simulink model "two_tanks_model_cascade"  (R2018b)
settings: Solver=FixedStepAuto  StartTime=0.0  StopTime=2400  FixedStep=0.1  RelTol=1e-3
model workspace (MATLAB code in the model file):
  | A1 = 1;
  | a1 = 0.1*0.1;
  | A2 = A1;
  | a2 = a1;
  | h10 = 1;
  | h20=1;
values from neighbouring files (symbols this model uses):
  K = yf/uf    (= 58.7333333333)    [two_tanks_cascade.m]    (also in two_tanks_cascade_ffwd.m)
  kc1 = 0.406    [two_tanks_cascade.m]    (also in two_tanks_cascade_ffwd.m)
  kc2 = 1    [two_tanks_cascade.m]    (also in two_tanks_cascade_ffwd.m)
  tau = 59    [two_tanks_cascade.m]    (also in two_tanks_cascade_ffwd.m)
  taui1 = t1/z1    (= 8.96)    [two_tanks_cascade.m]    (also in two_tanks_cascade_ffwd.m)
  taui2 = t2    (= 59)    [two_tanks_cascade.m]    (also in two_tanks_cascade_ffwd.m)
undefined symbols (not defined in the file or in its folder): theta
settings Model: PacingRate=100  Creator=kjartan  LastModifiedBy=kjartan

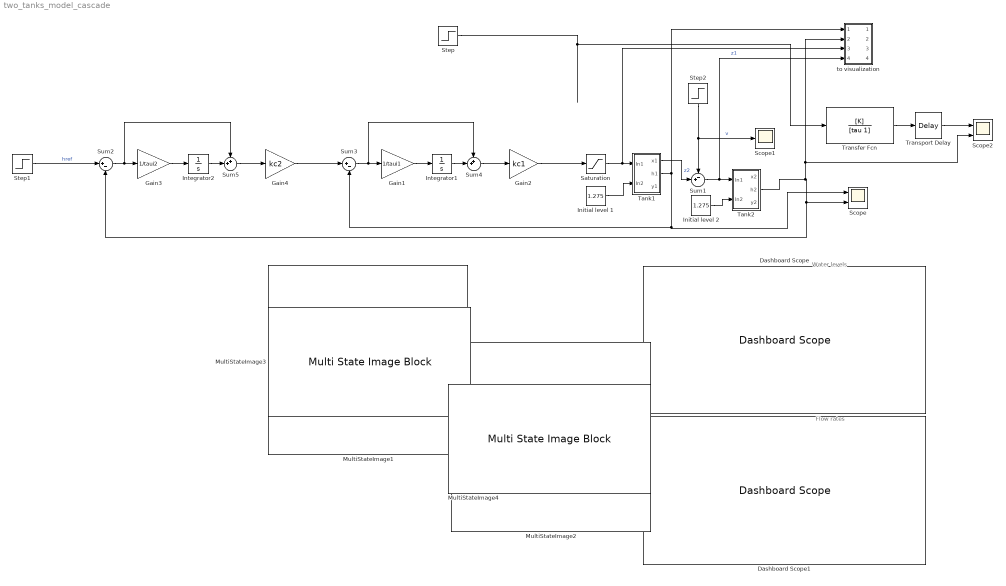
== system two_tanks_model_cascade ==
  note: Flow rates
  note: Water levels
  Dashboard Scope : DashboardScope  WebBlockId=50  Ymin=0  Ymax=2.6000000000000001
  Dashboard Scope1 : DashboardScope  WebBlockId=91  Ymin=0  Ymax=0.29999999999999999
  Gain1 : Gain  Gain=1/taui1
  Gain2 : Gain  Gain=kc1
  Gain3 : Gain  Gain=1/taui2
  Gain4 : Gain  Gain=kc2
  Initial level 1 : Constant  Value=1.275
  Initial level 2 : Constant  Value=1.275
  Integrator1 : Integrator
  Integrator2 : Integrator
  MultiStateImage1 : MultiStateImageBlock  WebBlockId=71
  MultiStateImage2 : MultiStateImageBlock  WebBlockId=119
  MultiStateImage3 : MultiStateImageBlock  WebBlockId=117  ScaleMode=Fill
  MultiStateImage4 : MultiStateImageBlock  WebBlockId=126  ScaleMode=Fill
  Saturation : Saturate  LowerLimit=0
  Scope : Scope  NumInputPorts=2
  Scope1 : Scope
  Scope2 : Scope  NumInputPorts=2
  Step : Step  Time=800  Before=0.05  After=0.065  SampleTime=0
  Step1 : Step  Time=800  Before=1.275  After=2  SampleTime=0
  Step2 : Step  Time=1400  After=0.015  SampleTime=0
  Sum1 : Sum  Inputs=-+|
  Sum2 : Sum  Inputs=|+-
  Sum3 : Sum  Inputs=|+-
  Sum4 : Sum  Inputs=++|
  Sum5 : Sum  Inputs=++|
  Tank1 : Subsystem
  Tank2 : Subsystem
  Transfer Fcn : TransferFcn  Numerator=[K]  Denominator=[tau 1]
  Transport Delay : TransportDelay  DelayTime=theta
  to visualization : Subsystem
  wires:
  Tank1/1(x1) -> Sum1/2  "z2"
  Tank1/2(h1) -> to visualization/1(In2), Sum3/2, Scope/1
  Sum1/1 -> to visualization/4(In4), Tank2/1(In1)
  Step1/1 -> Sum2/1  "href"
  Saturation/1 -> to visualization/3(In3), Tank1/1(In1)  "z1"
  Initial level 2/1 -> Tank2/2(In2)
  Initial level 1/1 -> Tank1/2(In2)
  Step2/1 -> Sum1/1, Scope1/1  "v"
  Step/1 -> Transfer Fcn/1
  Transfer Fcn/1 -> Transport Delay/1
  Transport Delay/1 -> Scope2/1
  Gain1/1 -> Integrator1/1
  Integrator1/1 -> Sum4/2
  Sum3/1 -> Sum4/1, Gain1/1
  Sum4/1 -> Gain2/1
  Gain2/1 -> Saturation/1
  Gain3/1 -> Integrator2/1
  Tank2/2(h2) -> Scope2/2, to visualization/2(In1), Sum2/2, Scope/2
  Gain4/1 -> Sum3/1
  Sum2/1 -> Sum5/1, Gain3/1
  Sum5/1 -> Gain4/1
  Integrator2/1 -> Sum5/2

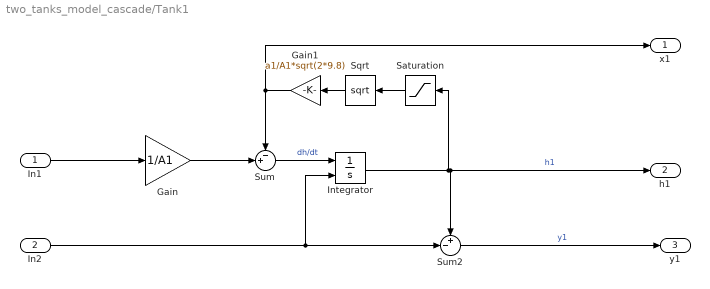
== system two_tanks_model_cascade/Tank1 ==
  In1 : Inport
  In2 : Inport  Port=2
  Gain : Gain  Gain=1/A1
  Gain1 : Gain  Gain=a1/A1*sqrt(2*9.8)
  Integrator : Integrator  InitialConditionSource=external  InitialCondition=h10
  Saturation : Saturate  UpperLimit=100  LowerLimit=0
  Sqrt : Sqrt  SaturateOnIntegerOverflow=on
  Sum : Sum  Inputs=-+|
  Sum2 : Sum  Inputs=+-|
  x1 : Outport
  h1 : Outport  Port=2
  y1 : Outport  Port=3
  wires:
  Gain1/1 -> x1/1, Sum/1
  Gain/1 -> Sum/2
  Sum/1 -> Integrator/1  "dh/dt"
  In1/1 -> Gain/1
  Sum2/1 -> y1/1  "y1"
  Sqrt/1 -> Gain1/1
  Integrator/1 -> Saturation/1, h1/1, Sum2/1  "h1"
  In2/1 -> Sum2/2, Integrator/2
  Saturation/1 -> Sqrt/1

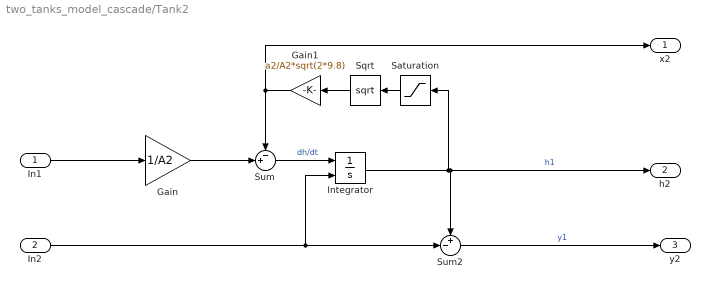
== system two_tanks_model_cascade/Tank2 ==
  In1 : Inport
  In2 : Inport  Port=2
  Gain : Gain  Gain=1/A2
  Gain1 : Gain  Gain=a2/A2*sqrt(2*9.8)
  Integrator : Integrator  InitialConditionSource=external  InitialCondition=h10
  Saturation : Saturate  UpperLimit=100  LowerLimit=0
  Sqrt : Sqrt  SaturateOnIntegerOverflow=on
  Sum : Sum  Inputs=-+|
  Sum2 : Sum  Inputs=+-|
  x2 : Outport
  h2 : Outport  Port=2
  y2 : Outport  Port=3
  wires:
  Gain1/1 -> x2/1, Sum/1
  Gain/1 -> Sum/2
  Sum/1 -> Integrator/1  "dh/dt"
  In1/1 -> Gain/1
  Sum2/1 -> y2/1  "y1"
  Sqrt/1 -> Gain1/1
  Integrator/1 -> Saturation/1, h2/1, Sum2/1  "h1"
  In2/1 -> Sum2/2, Integrator/2
  Saturation/1 -> Sqrt/1

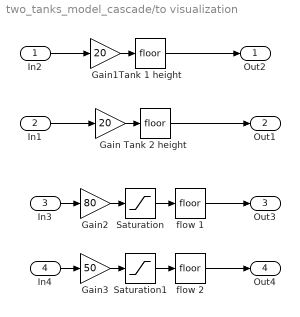
== system two_tanks_model_cascade/to visualization ==
  In2 : Inport
  In1 : Inport  Port=2
  In3 : Inport  Port=3
  In4 : Inport  Port=4
  Gain : Gain  Gain=20
  Gain1 : Gain  Gain=20
  Gain2 : Gain  Gain=80
  Gain3 : Gain  Gain=50
  Saturation : Saturate  UpperLimit=10  LowerLimit=0
  Saturation1 : Saturate  UpperLimit=5  LowerLimit=0
  Tank 1 height : Rounding
  Tank 2 height : Rounding
  flow 1 : Rounding
  flow 2 : Rounding
  Out2 : Outport
  Out1 : Outport  Port=2
  Out3 : Outport  Port=3
  Out4 : Outport  Port=4
  wires:
  Tank 2 height/1 -> Out1/1
  Gain/1 -> Tank 2 height/1
  In1/1 -> Gain/1
  Tank 1 height/1 -> Out2/1
  Gain1/1 -> Tank 1 height/1
  In2/1 -> Gain1/1
  flow 1/1 -> Out3/1
  Gain2/1 -> Saturation/1
  In3/1 -> Gain2/1
  flow 2/1 -> Out4/1
  In4/1 -> Gain3/1
  Gain3/1 -> Saturation1/1
  Saturation/1 -> flow 1/1
  Saturation1/1 -> flow 2/1
